simulink library "merge_activation_lib"  (Simulink 8.2)
settings: Solver=ode1  StartTime=0.0  StopTime=Inf  FixedStep=0.001  RelTol=1e-3
PostLoadFcn:
  | , if any(exist('dsrtsu_mdlpostloadfcn', 'file') == [2, 3, 6]), try dsrtsu_mdlpostloadfcn('Execute', bdroot); catch fprintf('Error in PostLoadFcn (dsrtsu_mdlpostloadfcn) for model "%s":\n %s\n', bdroot, lasterr); end, end,
undefined symbols (not defined in the file or in its folder): MergeStateEnum, VehicleRoleEnum
libraries: simulink x7, merge_activation_lib x4
settings Model: DSRTSU_INTERNAL_RTI_VER=450  DSRTSU_INTERNAL_RTI_TYPE=rti1401  DSRTSU_INTERNAL_RTIFPGA=40  Creator=rushk1  LastModifiedBy=rushk1

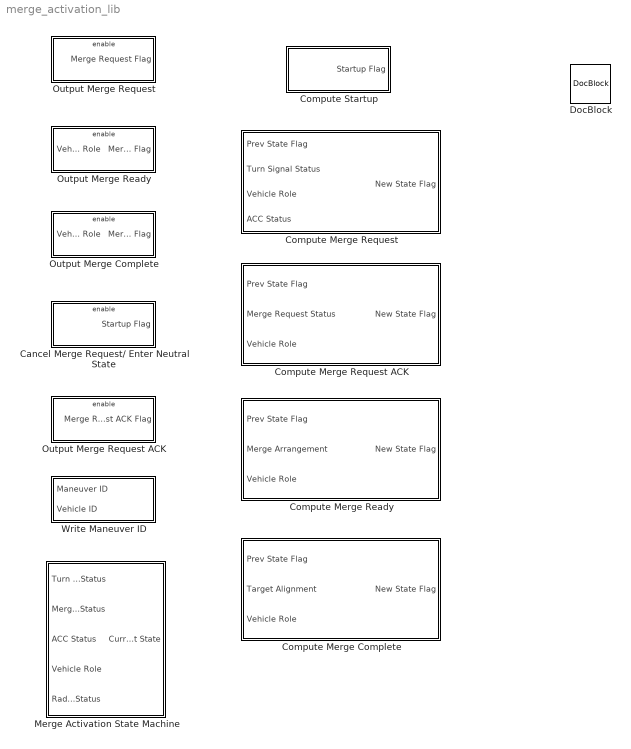
== system merge_activation_lib ==
  Cancel Merge Request/ Enter Neutral State : Subsystem
  Compute Merge Complete : Subsystem
  Compute Merge Ready : Subsystem
  Compute Merge Request : Subsystem
  Compute Merge Request ACK : Subsystem
  Compute Startup : Subsystem
  DocBlock : simulink/Model-Wide Utilities/DocBlock  DocumentType=Text
      content=|
      | This library is responsible for computing the state of each vehicle in the
      | experiment.
      |
      | The state computation is set up such all states are linear (state 2
      | requires meeting the requirements for state 2). As such each state block
      | takes in the information about its requirements and the previous state
      | block's output. If the requirements are met the block outputs the new
      | state. If they are not met the block outputs the previous state block's
      | value. This way requirements are computed sequentially and the highest
      | level that gets satisfied is the ultimate output at the end.
      |
      | The first state (0x00 - STARTUP) is output by the Compute Startup block as
      | a constant, thus making it the default.
      |
      | Compute Merge Request requires the the current vehicle role to be merge,
      | the vehicle to be in ACC, and the turn signal to be on (in either
      | direction).
      |
      | Compute Merge Request ACK requires the vehicle role to be follow, the merge
      | vehicle's and the merge vehicle's merge request to be on.
      |
      | Compute Merge Ready requires the previous state to be merge request or
      | merge request ack and for the Merge Arrangement input to be true. The merge
      | arrangement is computed by a separate block in the Lane Merge Control Code
      | but to summarize:
      |
      | For the merge vehicle the closest radar object must be at >=G distance from
      | the vehicle.
      |
      | For the follow vehicle the closest radar object must also be at >=G
      | distance from the vehicle and it must also have at least two radar targets.
      |
      | Compute Merge Complete requires the previous state to be merge ready and is
      | active when the target is aligned in the same lane (computed in a separate
      | block).
      |
      | In the Lane Merge Control Code, these 5 blocks are chained (output to input)
      | to produce the overall state value for the current timestep. This value is
      | recomputed every timestep, unless the latch is engaged. The latch is engaged
      | if the merge complete state has been held for 20 consecutive timesteps and
      | is cleared once the ACC system has been deactivated.
  Merge Activation State Machine : Subsystem
  Output Merge Complete : Subsystem
  Output Merge Ready : Subsystem
  Output Merge Request : Subsystem
  Output Merge Request ACK : Subsystem  TreatAsAtomicUnit=on
  Write Maneuver ID : Subsystem

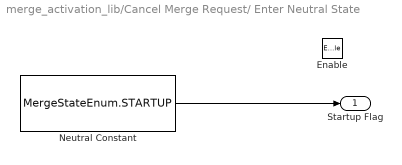
== system merge_activation_lib/Cancel Merge Request/ Enter Neutral State ==
  Enable : EnablePort
  Neutral Constant : Constant  Value=MergeStateEnum.STARTUP
  Startup Flag : Outport
  wires:
  Neutral Constant/1 -> Startup Flag/1

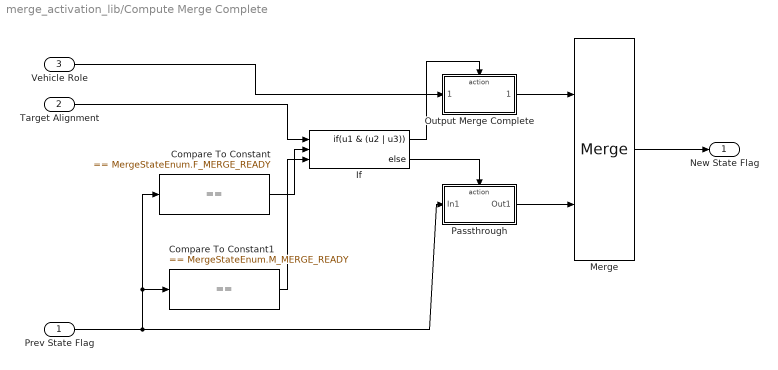
== system merge_activation_lib/Compute Merge Complete ==
  Prev State Flag : Inport
  Target Alignment : Inport  Port=2
  Vehicle Role : Inport  Port=3
  Compare To Constant : simulink/Logic and Bit Operations/Compare To Constant  relop===  const=MergeStateEnum.F_MERGE_READY  OutDataTypeStr=boolean
  Compare To Constant1 : simulink/Logic and Bit Operations/Compare To Constant  relop===  const=MergeStateEnum.M_MERGE_READY  OutDataTypeStr=boolean
  If : If  NumInputs=3  IfExpression=u1 & (u2 | u3)
  Merge : Merge
  Output Merge Complete : Subsystem  TreatAsAtomicUnit=on
  Passthrough : Subsystem  TreatAsAtomicUnit=on
  New State Flag : Outport
  wires:
  Compare To Constant/1 -> If/2
  Merge/1 -> New State Flag/1
  Output Merge Complete/1(Merge Complete) -> Merge/1
  Passthrough/1(Out1) -> Merge/2
  Prev State Flag/1 -> Compare To Constant/1, Compare To Constant1/1, Passthrough/1(In1)
  If/2 -> Passthrough/Action
  If/1 -> Output Merge Complete/Action
  Target Alignment/1 -> If/1
  Compare To Constant1/1 -> If/3
  Vehicle Role/1 -> Output Merge Complete/1(Vehicle Role)

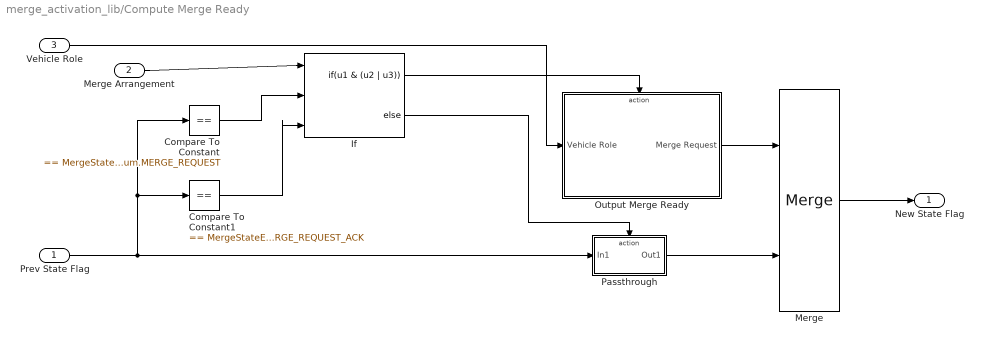
== system merge_activation_lib/Compute Merge Ready ==
  Prev State Flag : Inport
  Merge Arrangement : Inport  Port=2
  Vehicle Role : Inport  Port=3
  Compare To Constant : simulink/Logic and Bit Operations/Compare To Constant  relop===  const=MergeStateEnum.MERGE_REQUEST  OutDataTypeStr=boolean
  Compare To Constant1 : simulink/Logic and Bit Operations/Compare To Constant  relop===  const=MergeStateEnum.F_MERGE_REQUEST_ACK  OutDataTypeStr=boolean
  If : If  NumInputs=3  IfExpression=u1 & (u2 | u3)
  Merge : Merge
  Output Merge Ready : Subsystem  TreatAsAtomicUnit=on
  Passthrough : Subsystem  TreatAsAtomicUnit=on
  New State Flag : Outport
  wires:
  Merge Arrangement/1 -> If/1
  If/1 -> Output Merge Ready/Action
  If/2 -> Passthrough/Action
  Prev State Flag/1 -> Passthrough/1(In1), Compare To Constant/1, Compare To Constant1/1
  Passthrough/1(Out1) -> Merge/2
  Output Merge Ready/1(Merge Request) -> Merge/1
  Merge/1 -> New State Flag/1
  Compare To Constant/1 -> If/2
  Compare To Constant1/1 -> If/3
  Vehicle Role/1 -> Output Merge Ready/1(Vehicle Role)

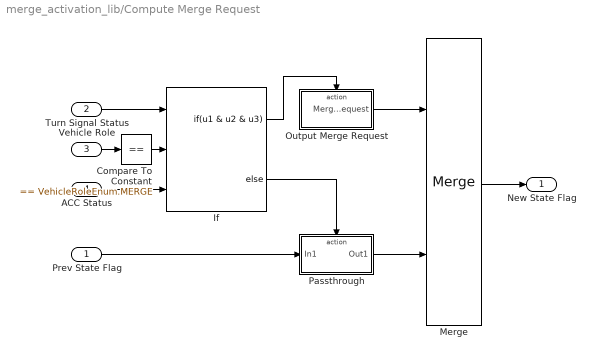
== system merge_activation_lib/Compute Merge Request ==
  Prev State Flag : Inport
  Turn Signal Status : Inport  Port=2
  Vehicle Role : Inport  Port=3
  ACC Status : Inport  Port=4
  Compare To Constant : simulink/Logic and Bit Operations/Compare To Constant  relop===  const=VehicleRoleEnum.MERGE  OutDataTypeStr=boolean
  If : If  NumInputs=3  IfExpression=u1 & u2 & u3
  Merge : Merge
  Output Merge Request : Subsystem  TreatAsAtomicUnit=on
  Passthrough : Subsystem  TreatAsAtomicUnit=on
  New State Flag : Outport
  wires:
  Turn Signal Status/1 -> If/1
  If/1 -> Output Merge Request/Action
  If/2 -> Passthrough/Action
  Vehicle Role/1 -> Compare To Constant/1
  Prev State Flag/1 -> Passthrough/1(In1)
  Passthrough/1(Out1) -> Merge/2
  Output Merge Request/1(Merge Request) -> Merge/1
  Merge/1 -> New State Flag/1
  ACC Status/1 -> If/3
  Compare To Constant/1 -> If/2

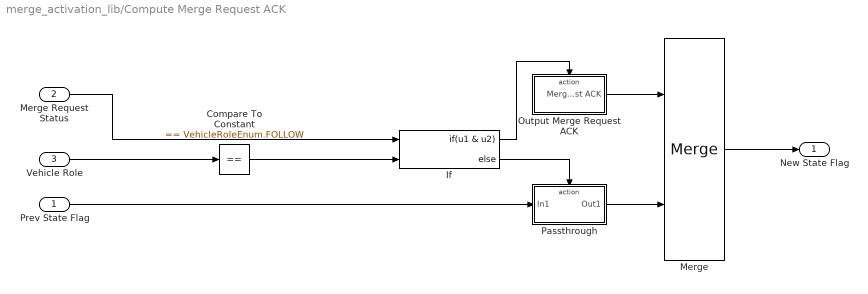
== system merge_activation_lib/Compute Merge Request ACK ==
  Prev State Flag : Inport
  Merge Request Status : Inport  Port=2
  Vehicle Role : Inport  Port=3
  Compare To Constant : simulink/Logic and Bit Operations/Compare To Constant  relop===  const=VehicleRoleEnum.FOLLOW  OutDataTypeStr=boolean
  If : If  NumInputs=2  IfExpression=u1 & u2
  Merge : Merge
  Output Merge Request ACK : Subsystem  TreatAsAtomicUnit=on
  Passthrough : Subsystem  TreatAsAtomicUnit=on
  New State Flag : Outport
  wires:
  Merge/1 -> New State Flag/1
  Output Merge Request ACK/1(Merge Request ACK) -> Merge/1
  Passthrough/1(Out1) -> Merge/2
  Prev State Flag/1 -> Passthrough/1(In1)
  If/2 -> Passthrough/Action
  If/1 -> Output Merge Request ACK/Action
  Merge Request Status/1 -> If/1
  Vehicle Role/1 -> Compare To Constant/1
  Compare To Constant/1 -> If/2

== system merge_activation_lib/Compute Startup ==
  Constant : Constant  Value=MergeStateEnum.STARTUP
  Startup Flag : Outport
  wires:
  Constant/1 -> Startup Flag/1

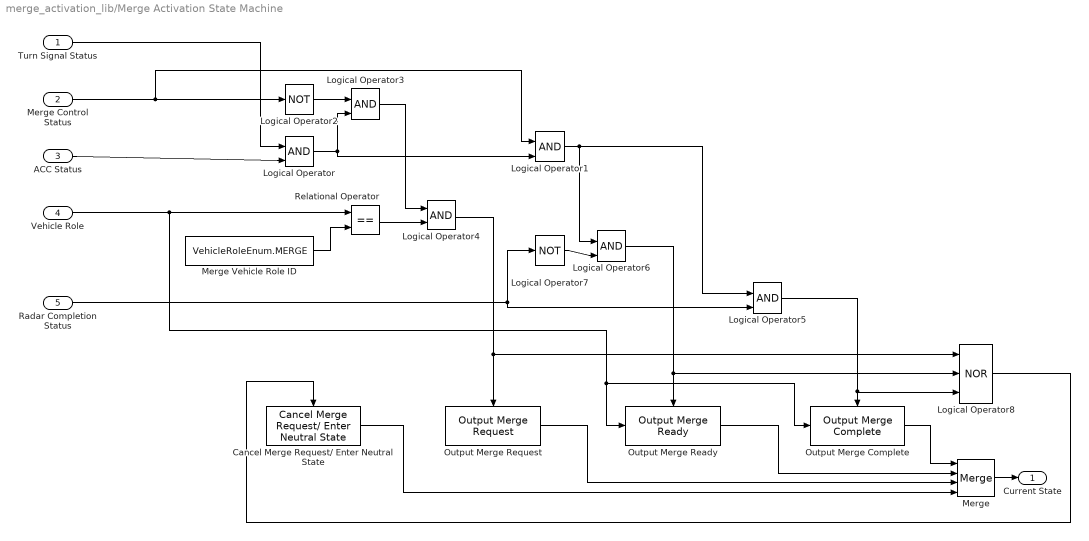
== system merge_activation_lib/Merge Activation State Machine ==
  Turn Signal Status : Inport
  Merge Control Status : Inport  Port=2
  ACC Status : Inport  Port=3
  Vehicle Role : Inport  Port=4
  Radar Completion Status : Inport  Port=5
  Cancel Merge Request/ Enter Neutral State : merge_activation_lib/Cancel Merge Request// Enter Neutral State
  Logical Operator{,1,3,5..6} (5 alike) : Logic  IconShape=distinctive  AllPortsSameDT=off  OutDataTypeStr=boolean
  Logical Operator2 : Logic  Operator=NOT  IconShape=distinctive  AllPortsSameDT=off  OutDataTypeStr=boolean
  Logical Operator4 : Logic  AllPortsSameDT=off  OutDataTypeStr=boolean
  Logical Operator7 : Logic  Operator=NOT  IconShape=distinctive  AllPortsSameDT=off  OutDataTypeStr=boolean
  Logical Operator8 : Logic  Operator=NOR  Inputs=3  IconShape=distinctive  AllPortsSameDT=off  OutDataTypeStr=boolean
  Merge : Merge  Inputs=4
  "Merge Vehicle Role ID " : Constant  Value=VehicleRoleEnum.MERGE
  Output Merge Complete : merge_activation_lib/Output Merge Complete
  Output Merge Ready : merge_activation_lib/Output Merge Ready
  Output Merge Request : merge_activation_lib/Output Merge Request
  Relational Operator : RelationalOperator  Operator===  OutDataTypeStr=boolean
  Current State : Outport
  wires:
  Vehicle Role/1 -> Output Merge Complete/1, Output Merge Ready/1, Relational Operator/1
  Turn Signal Status/1 -> Logical Operator/1
  Merge Control Status/1 -> Logical Operator1/1, Logical Operator2/1
  ACC Status/1 -> Logical Operator/2
  Logical Operator1/1 -> Logical Operator5/1, Logical Operator6/1
  Logical Operator2/1 -> Logical Operator3/1
  Logical Operator/1 -> Logical Operator1/2, Logical Operator3/2
  "Merge Vehicle Role ID "/1 -> Relational Operator/2
  Relational Operator/1 -> Logical Operator4/2
  Logical Operator3/1 -> Logical Operator4/1
  Logical Operator4/1 -> Output Merge Request/Enable, Logical Operator8/1
  Radar Completion Status/1 -> Logical Operator5/2, Logical Operator7/1
  Logical Operator5/1 -> Logical Operator8/3, Output Merge Complete/Enable
  Logical Operator7/1 -> Logical Operator6/2
  Logical Operator6/1 -> Logical Operator8/2, Output Merge Ready/Enable
  Cancel Merge Request/ Enter Neutral State/1 -> Merge/4
  Output Merge Request/1 -> Merge/3
  Output Merge Ready/1 -> Merge/2
  Output Merge Complete/1 -> Merge/1
  Merge/1 -> Current State/1
  Logical Operator8/1 -> Cancel Merge Request/ Enter Neutral State/Enable

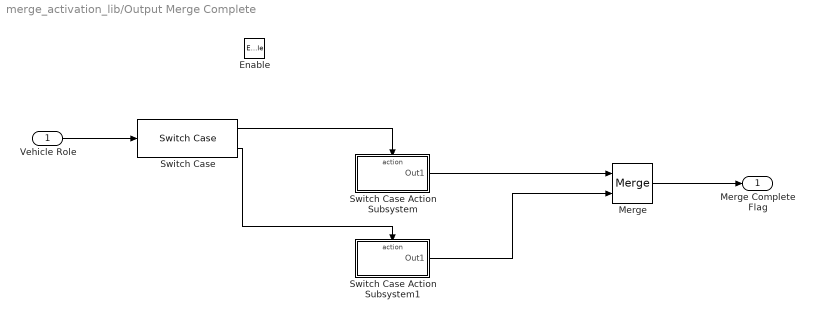
== system merge_activation_lib/Output Merge Complete ==
  "Vehicle Role " : Inport
  Enable : EnablePort
  Merge : Merge
  Switch Case : SwitchCase  CaseConditions={VehicleRoleEnum.MERGE, VehicleRoleEnum.FOLLOW}  ShowDefaultCase=off
  Switch Case Action Subsystem : Subsystem  AncestorBlock=merge_activation_lib/Output Merge Ready/Switch Case Action Subsystem  TreatAsAtomicUnit=on
  Switch Case Action Subsystem1 : Subsystem  AncestorBlock=merge_activation_lib/Output Merge Ready/Switch Case Action Subsystem1  TreatAsAtomicUnit=on
  Merge Complete Flag : Outport
  wires:
  Switch Case/1 -> Switch Case Action Subsystem/Action
  Switch Case/2 -> Switch Case Action Subsystem1/Action
  "Vehicle Role "/1 -> Switch Case/1
  Switch Case Action Subsystem/1(Out1) -> Merge/1
  Switch Case Action Subsystem1/1(Out1) -> Merge/2
  Merge/1 -> Merge Complete Flag/1

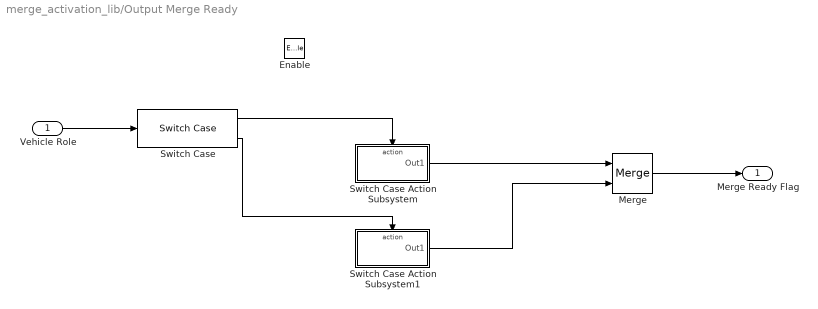
== system merge_activation_lib/Output Merge Ready ==
  "Vehicle Role " : Inport
  Enable : EnablePort
  Merge : Merge
  Switch Case : SwitchCase  CaseConditions={VehicleRoleEnum.MERGE, VehicleRoleEnum.FOLLOW}  ShowDefaultCase=off
  Switch Case Action Subsystem : Subsystem  TreatAsAtomicUnit=on
  Switch Case Action Subsystem1 : Subsystem  AncestorBlock=merge_activation_lib/Output Merge Ready/Switch Case Action Subsystem  TreatAsAtomicUnit=on
  Merge Ready Flag : Outport
  wires:
  Switch Case/1 -> Switch Case Action Subsystem/Action
  Switch Case/2 -> Switch Case Action Subsystem1/Action
  "Vehicle Role "/1 -> Switch Case/1
  Switch Case Action Subsystem/1(Out1) -> Merge/1
  Switch Case Action Subsystem1/1(Out1) -> Merge/2
  Merge/1 -> Merge Ready Flag/1

== system merge_activation_lib/Output Merge Request ==
  Enable : EnablePort
  Merge Request Constant : Constant  Value=MergeStateEnum.MERGE_REQUEST
  Merge Request Flag : Outport
  wires:
  Merge Request Constant/1 -> Merge Request Flag/1

== system merge_activation_lib/Output Merge Request ACK ==
  Enable : EnablePort
  Constant : Constant  Value=MergeStateEnum.MERGE_REQUEST_ACK
  Merge Request ACK Flag : Outport
  wires:
  Constant/1 -> Merge Request ACK Flag/1

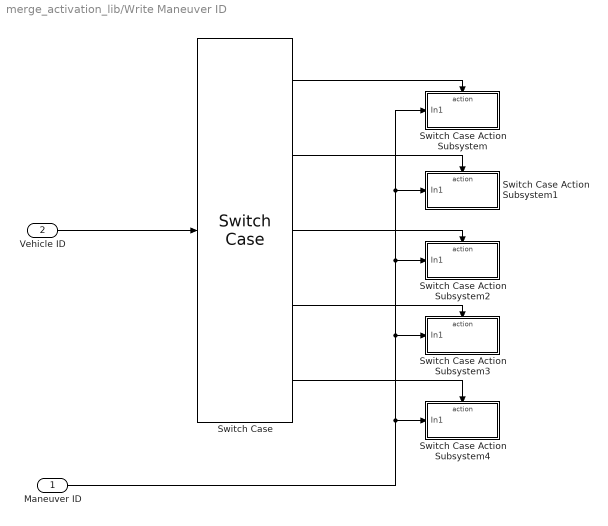
== system merge_activation_lib/Write Maneuver ID ==
  Maneuver ID : Inport
  Vehicle ID : Inport  Port=2
  Switch Case : SwitchCase  CaseConditions={1,2,3,4,5}  ShowDefaultCase=off
  Switch Case Action Subsystem : Subsystem  TreatAsAtomicUnit=on
  Switch Case Action Subsystem1 : Subsystem  TreatAsAtomicUnit=on
  Switch Case Action Subsystem2 : Subsystem  TreatAsAtomicUnit=on
  Switch Case Action Subsystem3 : Subsystem  TreatAsAtomicUnit=on
  Switch Case Action Subsystem4 : Subsystem  TreatAsAtomicUnit=on
  wires:
  Switch Case/5 -> Switch Case Action Subsystem4/Action
  Switch Case/4 -> Switch Case Action Subsystem3/Action
  Switch Case/3 -> Switch Case Action Subsystem2/Action
  Switch Case/2 -> Switch Case Action Subsystem1/Action
  Switch Case/1 -> Switch Case Action Subsystem/Action
  Vehicle ID/1 -> Switch Case/1
  Maneuver ID/1 -> Switch Case Action Subsystem/1(In1), Switch Case Action Subsystem1/1(In1), Switch Case Action Subsystem2/1(In1), Switch Case Action Subsystem3/1(In1), Switch Case Action Subsystem4/1(In1)

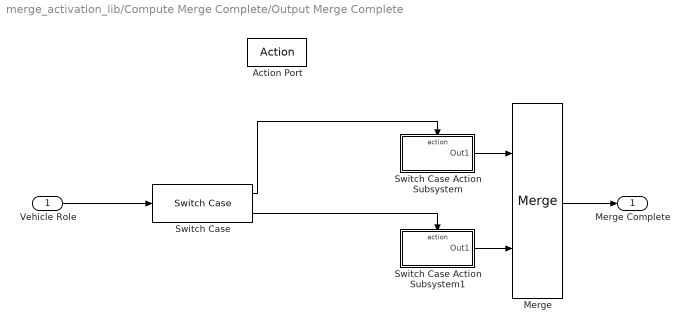
== system merge_activation_lib/Compute Merge Complete/Output Merge Complete ==
  Vehicle Role : Inport
  Action Port : ActionPort
  Merge : Merge
  Switch Case : SwitchCase  CaseConditions={VehicleRoleEnum.MERGE, VehicleRoleEnum.FOLLOW}  ShowDefaultCase=off
  Switch Case Action Subsystem : Subsystem  AncestorBlock=merge_activation_lib/Compute Merge Ready/Output Merge Ready/Switch Case Action Subsystem  TreatAsAtomicUnit=on
  Switch Case Action Subsystem1 : Subsystem  AncestorBlock=merge_activation_lib/Compute Merge Ready/Output Merge Ready/Switch Case Action Subsystem1  TreatAsAtomicUnit=on
  Merge Complete : Outport
  wires:
  Switch Case/1 -> Switch Case Action Subsystem/Action
  Switch Case/2 -> Switch Case Action Subsystem1/Action
  Switch Case Action Subsystem/1(Out1) -> Merge/1
  Switch Case Action Subsystem1/1(Out1) -> Merge/2
  Merge/1 -> Merge Complete/1
  Vehicle Role/1 -> Switch Case/1

== system merge_activation_lib/Compute Merge Complete/Passthrough ==
  In1 : Inport
  Action Port : ActionPort
  Out1 : Outport
  wires:
  In1/1 -> Out1/1

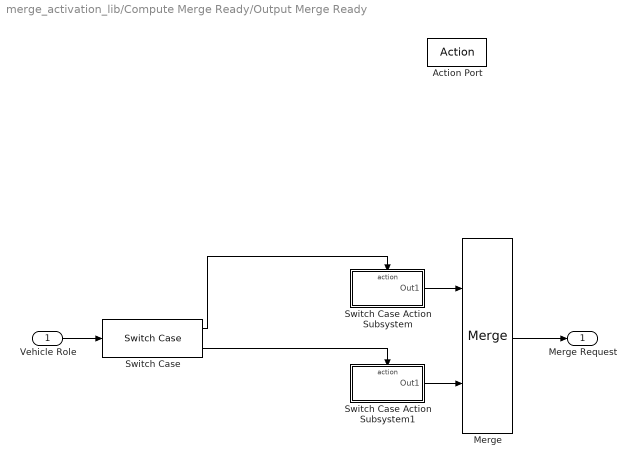
== system merge_activation_lib/Compute Merge Ready/Output Merge Ready ==
  Vehicle Role : Inport
  Action Port : ActionPort
  Merge : Merge
  Switch Case : SwitchCase  CaseConditions={VehicleRoleEnum.MERGE, VehicleRoleEnum.FOLLOW}  ShowDefaultCase=off
  Switch Case Action Subsystem : Subsystem  TreatAsAtomicUnit=on
  Switch Case Action Subsystem1 : Subsystem  TreatAsAtomicUnit=on
  Merge Request : Outport
  wires:
  Switch Case/1 -> Switch Case Action Subsystem/Action
  Switch Case/2 -> Switch Case Action Subsystem1/Action
  Vehicle Role/1 -> Switch Case/1
  Switch Case Action Subsystem/1(Out1) -> Merge/1
  Switch Case Action Subsystem1/1(Out1) -> Merge/2
  Merge/1 -> Merge Request/1

== system merge_activation_lib/Compute Merge Ready/Passthrough ==
  In1 : Inport
  Action Port : ActionPort
  Out1 : Outport
  wires:
  In1/1 -> Out1/1

== system merge_activation_lib/Compute Merge Request/Output Merge Request ==
  Action Port : ActionPort  ActionType=then
  Constant : Constant  Value=MergeStateEnum.MERGE_REQUEST
  Merge Request : Outport
  wires:
  Constant/1 -> Merge Request/1

== system merge_activation_lib/Compute Merge Request/Passthrough ==
  In1 : Inport
  Action Port : ActionPort  ActionType=else
  Out1 : Outport
  wires:
  In1/1 -> Out1/1

== system merge_activation_lib/Compute Merge Request ACK/Output Merge Request ACK ==
  Action Port : ActionPort
  Constant : Constant  Value=MergeStateEnum.F_MERGE_REQUEST_ACK
  Merge Request ACK : Outport
  wires:
  Constant/1 -> Merge Request ACK/1

== system merge_activation_lib/Compute Merge Request ACK/Passthrough ==
  In1 : Inport
  Action Port : ActionPort
  Out1 : Outport
  wires:
  In1/1 -> Out1/1

== system merge_activation_lib/Output Merge Complete/Switch Case Action Subsystem ==
  Action Port : ActionPort
  Constant : Constant  Value=MergeStateEnum.M_MERGE_COMPLETE
  Out1 : Outport
  wires:
  Constant/1 -> Out1/1

== system merge_activation_lib/Output Merge Complete/Switch Case Action Subsystem1 ==
  Action Port : ActionPort
  Merge Ready Constant : Constant  Value=MergeStateEnum.F_MERGE_COMPLETE
  Out1 : Outport
  wires:
  Merge Ready Constant/1 -> Out1/1

== system merge_activation_lib/Output Merge Ready/Switch Case Action Subsystem ==
  Action Port : ActionPort  ActionType=case
  Constant : Constant  Value=MergeStateEnum.M_MERGE_READY
  Out1 : Outport
  wires:
  Constant/1 -> Out1/1

== system merge_activation_lib/Output Merge Ready/Switch Case Action Subsystem1 ==
  Action Port : ActionPort
  Merge Ready Constant : Constant  Value=MergeStateEnum.F_MERGE_READY
  Out1 : Outport
  wires:
  Merge Ready Constant/1 -> Out1/1

== system merge_activation_lib/Write Maneuver ID/Switch Case Action Subsystem ==
  In1 : Inport
  Action Port : ActionPort
  Data Store Write : DataStoreWrite  DataStoreName=BSMStoreSignal  DataStoreElements=BSMStoreSignal.Veh1BSM.vehManID
  wires:
  In1/1 -> Data Store Write/1

== system merge_activation_lib/Write Maneuver ID/Switch Case Action Subsystem1 ==
  In1 : Inport
  Action Port : ActionPort
  Data Store Write : DataStoreWrite  DataStoreName=BSMStoreSignal  DataStoreElements=BSMStoreSignal.Veh2BSM.vehManID
  wires:
  In1/1 -> Data Store Write/1

== system merge_activation_lib/Write Maneuver ID/Switch Case Action Subsystem2 ==
  In1 : Inport
  Action Port : ActionPort
  Data Store Write : DataStoreWrite  DataStoreName=BSMStoreSignal  DataStoreElements=BSMStoreSignal.Veh3BSM.vehManID
  wires:
  In1/1 -> Data Store Write/1

== system merge_activation_lib/Write Maneuver ID/Switch Case Action Subsystem3 ==
  In1 : Inport
  Action Port : ActionPort
  Data Store Write : DataStoreWrite  DataStoreName=BSMStoreSignal  DataStoreElements=BSMStoreSignal.Veh4BSM.vehManID
  wires:
  In1/1 -> Data Store Write/1

== system merge_activation_lib/Write Maneuver ID/Switch Case Action Subsystem4 ==
  In1 : Inport
  Action Port : ActionPort
  Data Store Write : DataStoreWrite  DataStoreName=BSMStoreSignal  DataStoreElements=BSMStoreSignal.Veh5BSM.vehManID
  wires:
  In1/1 -> Data Store Write/1

== system merge_activation_lib/Compute Merge Complete/Output Merge Complete/Switch Case Action Subsystem ==
  Action Port : ActionPort
  Constant : Constant  Value=MergeStateEnum.M_MERGE_COMPLETE
  Out1 : Outport
  wires:
  Constant/1 -> Out1/1

== system merge_activation_lib/Compute Merge Complete/Output Merge Complete/Switch Case Action Subsystem1 ==
  Action Port : ActionPort
  Constant : Constant  Value=MergeStateEnum.F_MERGE_COMPLETE
  Out1 : Outport
  wires:
  Constant/1 -> Out1/1

== system merge_activation_lib/Compute Merge Ready/Output Merge Ready/Switch Case Action Subsystem ==
  Action Port : ActionPort  ActionType=case
  Constant : Constant  Value=MergeStateEnum.M_MERGE_READY
  Out1 : Outport
  wires:
  Constant/1 -> Out1/1

== system merge_activation_lib/Compute Merge Ready/Output Merge Ready/Switch Case Action Subsystem1 ==
  Action Port : ActionPort  ActionType=case
  Constant : Constant  Value=MergeStateEnum.F_MERGE_READY
  Out1 : Outport
  wires:
  Constant/1 -> Out1/1
